simulink model "Plant"  (R2023b)
settings: Solver=VariableStepAuto  StartTime=0.0  StopTime=10.0  RelTol=1e-3
values from neighbouring files (symbols this model uses):
  Force_Applied = [0 0 0]    [init_plant.m]
  g = 0    [init_plant.m]
  Inertia = [ 1 0 0 ... (first row only)    [init_plant.m]
  Initial_Pos = [0 5 0]    [init_plant.m]
  m = 1    [init_plant.m]
  Moments = [0 0 0]    [init_plant.m]
  pqr_0 = [0 0 0]'    [init_plant.m]
  q_0 = Euler_To_Quaternion_ScalarFirst(Euler_Initial)'    [init_plant.m]
libraries: simulink x1, matrix_library x1, aerolibutil x1, aerolibanimutils x1, vrlib x1
settings Model: Creator=benjackson  LastModifiedBy=benjackson
settings OptimizationCC: ReuseModelBlockBuffer=off

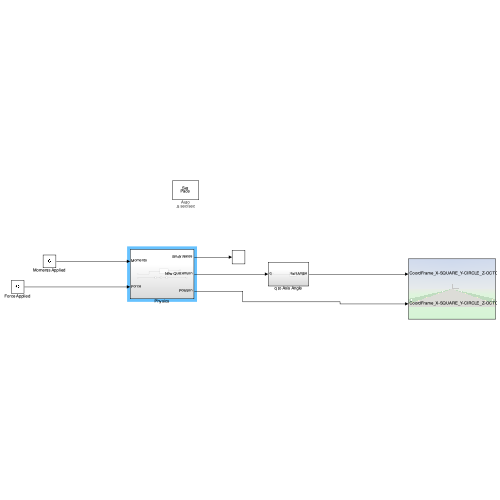
[thumbnail: Simulink's stored preview of the top-level diagram]
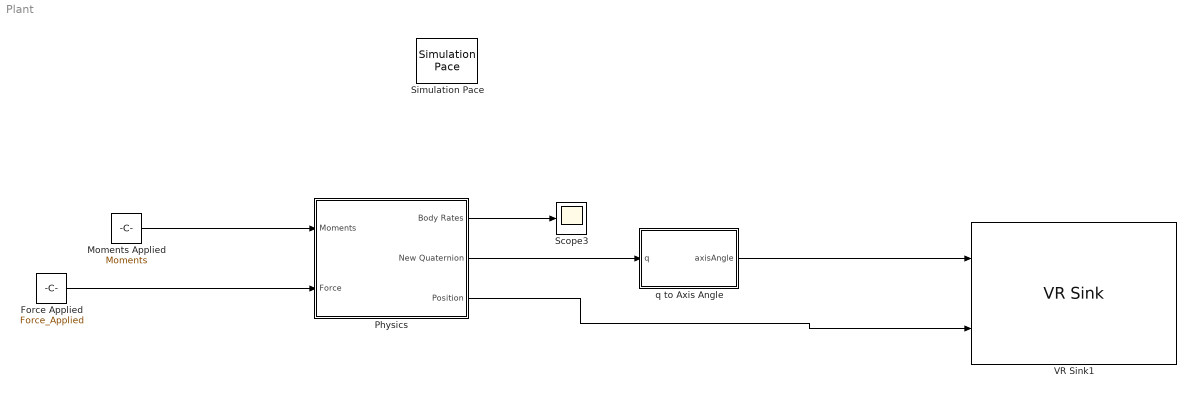
== system Plant ==
  Force Applied : Constant  Value=Force_Applied
  Moments Applied : Constant  Value=Moments
  Physics : Subsystem
  Scope3 : Scope
  Simulation Pace : aerolibanimutils/Simulation Pace  SimulationPace=.5  SleepMode=Auto  OutputPaceError=off  SampleTime=1/30
  VR Sink1 : vrlib/VR Sink  InstantiateOnLoad=on  SampleTime=0.1  ViewEnable=on  RemoteChange=off  RemoteView=off  FieldsWritten=CoordFrame_X-SQUARE_Y-CIRCLE_Z-OCTOGO_Transform.rotation.4.1.1.double#CoordFrame_X-SQUARE_Y-CIRCLE_Z-OCTOGO_Transform.translation.3.1.1.double  WorldFileName=World/World_RXN_WHL.x3d  WorldDescription=Straight Road Strip - 2 Lanes  AutoView=off  VideoDimensions=[]  AllowVariableSize=off
  q to Axis Angle : Subsystem
  wires:
  q to Axis Angle/1(axisAngle) -> VR Sink1/1
  Moments Applied/1 -> Physics/1(Moments)
  Force Applied/1 -> Physics/2(Force)
  Physics/1(Body Rates) -> Scope3/1
  Physics/2(New Quaternion) -> q to Axis Angle/1(q)
  Physics/3(Position) -> VR Sink1/2

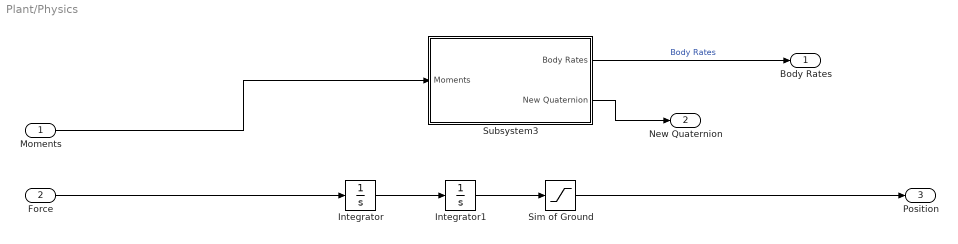
== system Plant/Physics ==
  Moments : Inport
  Force : Inport  Port=2
  Integrator : Integrator  InitialCondition=[0,m*g,0]  LimitOutput=on
  Integrator1 : Integrator  InitialCondition=Initial_Pos
  Sim of Ground : Saturate  UpperLimit=[200,200,200]  LowerLimit=[-200,0,-200]
  Subsystem3 : Subsystem
  Body Rates : Outport
  New Quaternion : Outport  Port=2
  Position : Outport  Port=3
  wires:
  Sim of Ground/1 -> Position/1
  Subsystem3/1(Body Rates) -> Body Rates/1  "Body Rates"
  Moments/1 -> Subsystem3/1(Moments)
  Force/1 -> Integrator/1
  Integrator1/1 -> Sim of Ground/1
  Subsystem3/2(New Quaternion) -> New Quaternion/1
  Integrator/1 -> Integrator1/1

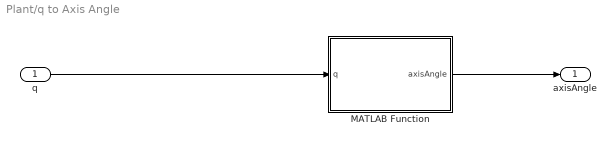
== system Plant/q to Axis Angle ==
  q : Inport
  MATLAB Function : MATLAB Function  TreatAsAtomicUnit=on
  axisAngle : Outport
  wires:
  q/1 -> MATLAB Function/1(q)
  MATLAB Function/1(axisAngle) -> axisAngle/1

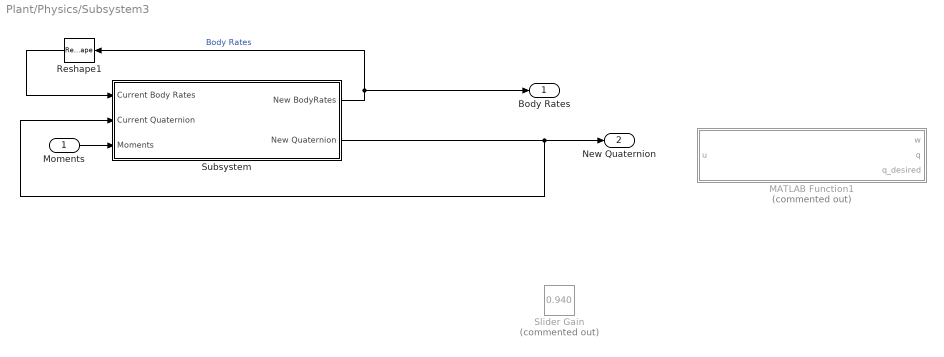
== system Plant/Physics/Subsystem3 ==
  Moments : Inport
  MATLAB Function1 : MATLAB Function  Commented=on  TreatAsAtomicUnit=on
  Reshape1 : Reshape  OutputDimensionality=Customize  OutputDimensions=[1,3]
  Slider Gain : simulink/Math Operations/Slider Gain  Commented=on  gain=0.940  low=0  high=2
  Subsystem : Subsystem
  Body Rates : Outport
  New Quaternion : Outport  Port=2
  wires:
  Subsystem/1(New BodyRates) -> Reshape1/1, Body Rates/1  "Body Rates"
  Subsystem/2(New Quaternion) -> Subsystem/2(Current Quaternion), New Quaternion/1
  Moments/1 -> Subsystem/3(Moments)
  Reshape1/1 -> Subsystem/1(Current Body Rates)

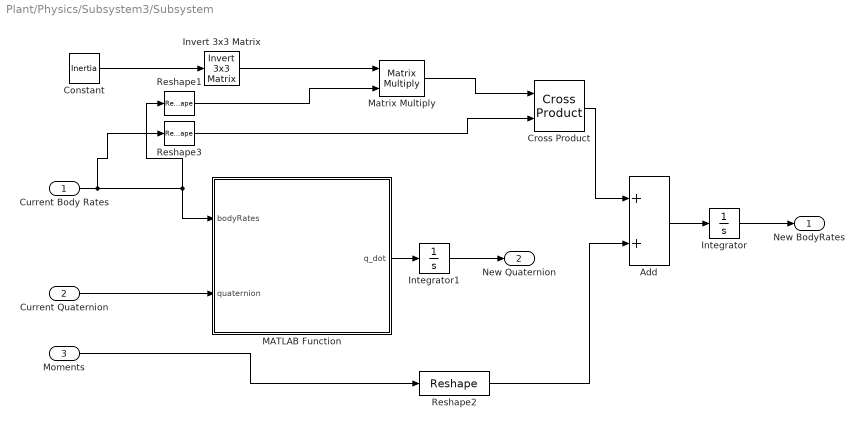
== system Plant/Physics/Subsystem3/Subsystem ==
  Current Body Rates : Inport
  Current Quaternion : Inport  Port=2
  Moments : Inport  Port=3
  Add : Sum
  Constant : Constant  Value=Inertia
  Cross Product : matrix_library/Cross Product
  Integrator : Integrator  InitialCondition=pqr_0
  Integrator1 : Integrator  InitialCondition=q_0
  Invert 3x3 Matrix : aerolibutil/Invert  3x3 Matrix
  MATLAB Function : MATLAB Function  TreatAsAtomicUnit=on
  Matrix Multiply : Product  Multiplication=Matrix(*)
  Reshape1 : Reshape  OutputDimensionality=Customize  OutputDimensions=[3,1]
  Reshape2 : Reshape  OutputDimensionality=Customize  OutputDimensions=[3,1]
  Reshape3 : Reshape  OutputDimensionality=Customize  OutputDimensions=[3,1]
  New BodyRates : Outport
  New Quaternion : Outport  Port=2
  wires:
  Matrix Multiply/1 -> Cross Product/1
  Current Quaternion/1 -> MATLAB Function/2(quaternion)
  Integrator/1 -> New BodyRates/1
  Constant/1 -> Invert 3x3 Matrix/1
  MATLAB Function/1(q_dot) -> Integrator1/1
  Integrator1/1 -> New Quaternion/1
  Current Body Rates/1 -> MATLAB Function/1(bodyRates), Reshape1/1, Reshape3/1
  Invert 3x3 Matrix/1 -> Matrix Multiply/1
  Cross Product/1 -> Add/1
  Add/1 -> Integrator/1
  Moments/1 -> Reshape2/1
  Reshape3/1 -> Cross Product/2
  Reshape1/1 -> Matrix Multiply/2
  Reshape2/1 -> Add/2

== matlab function Plant/Physics/Subsystem3/MATLAB Function1 ==
  data: w input; q input; u output; q_desired input
 function u = control(w,q,q_desired)
    
    q_current = q;

    wx = w(1);
    wy = w(2);
    wz = w(3);

    qe = [    q_desired(1),  q_desired(2),  q_desired(3),  q_desired(4);...
             -q_desired(2),  q_desired(1),  q_desired(4), -q_desired(3);...
             -q_desired(3), -q_desired(4),  q_desired(1),  q_desired(2);...
             -q_desired(4),  q_desired(3), -q_desired(2),  q_desired(1)]*q_current;
    
    u = [-30*wx-40*qe(2); -50*wy-30*qe(3); -50*wz-30*qe(4) ];

end

== matlab function Plant/Physics/Subsystem3/Subsystem/MATLAB Function ==
  data: bodyRates input; quaternion input; q_dot output
function q_dot = getBodyRates(bodyRates,quaternion)

    p = bodyRates(1);
    q = bodyRates(2); 
    r = bodyRates(3);
    
    half_Q_Matrix =   0.5 * [  0, -p, -q, -r
                               p,  0,  r, -q
                               q, -r,  0,  p
                               r,  q, -p,  0];
                
    qVec  =  [quaternion(1); quaternion(2); quaternion(3); quaternion(4)];
    q_dot =  (half_Q_Matrix * qVec);     
    
end

== matlab function Plant/q to Axis Angle/MATLAB Function ==
  data: q input; axisAngle output

function axisAngle = Quaternion_To_AxisAngle(q)
    for  i = 1:4
        if q(i) > 1 
            q(i) = 1.0;
            disp(q)
        end
    end

    qw = q(1);
    qx = q(2);
    qy = q(3);
    qz = q(4);
  

    theta = 2*acos(qw);

    if theta == 0 
        x = 1;
        y = 0;
        z = 0;
    else
        x = qx/(sin(theta/2));
        y = qy/(sin(theta/2));
        z = qz/(sin(theta/2));
    end
    
    %Vector comes first in our axis representation and angle comes last
    axisAngle = [x,z,y,theta];

end
